simulink model "rc_filter_test"  (R2020b)
settings: Solver=VariableStepAuto  StartTime=0.0  StopTime=10.0  RelTol=1e-3
undefined symbols (not defined in the file): C, current_gain, R, R_load, R_sense
libraries: fl_lib x7, nesl_utility x4, ee_lib x1
settings Model: Creator=akern  LastModifiedBy=akern

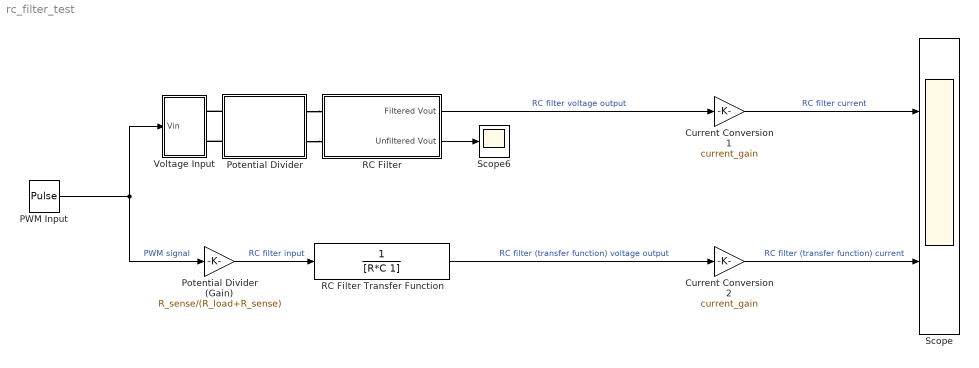
== system rc_filter_test ==
  Current Conversion 1 : Gain  Gain=current_gain
  Current Conversion 2 : Gain  Gain=current_gain
  PWM Input : DiscretePulseGenerator  PulseType=Time based  Amplitude=5  Period=1/500  PulseWidth=50
  Potential Divider : Subsystem
  Potential Divider (Gain) : Gain  Gain=R_sense/(R_load+R_sense)
  RC Filter : Subsystem
  RC Filter Transfer Function : TransferFcn  Numerator=[0 1]  Denominator=[R*C 1]
  Scope : Scope  NumInputPorts=2
  Scope6 : Scope
  Voltage Input : Subsystem
  wires:
  Current Conversion 1/1 -> Scope/1  "RC filter current"
  RC Filter/1(Filtered Vout) -> Current Conversion 1/1  "RC filter voltage output"
  RC Filter Transfer Function/1 -> Current Conversion 2/1  "RC filter (transfer function) voltage output"
  Potential Divider (Gain)/1 -> RC Filter Transfer Function/1  "RC filter input"
  PWM Input/1 -> Potential Divider (Gain)/1, Voltage Input/1(Vin)  "PWM signal"
  Current Conversion 2/1 -> Scope/2  "RC filter (transfer function) current"
  RC Filter/2(Unfiltered Vout) -> Scope6/1
  connections:
  Potential Divider/RConn2 -- RC Filter/LConn2
  Potential Divider/LConn2 -- Voltage Input/RConn2
  Potential Divider/LConn1 -- Voltage Input/RConn1
  Potential Divider/RConn1 -- RC Filter/LConn1

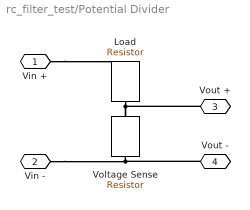
== system rc_filter_test/Potential Divider ==
  Load : fl_lib/Electrical/Electrical Elements/Resistor  R=R_load Ohm  i_specify=off  i_priority=None  i=0 A  i_nominal_specify=off  i_nominal_unit=A  i_nominal_value=1  v_specify=off  v_priority=None  v=0 V  v_nominal_specify=off  v_nominal_unit=V  v_nominal_value=1
  Voltage Sense : fl_lib/Electrical/Electrical Elements/Resistor  R=1 Ohm  i_specify=off  i_priority=None  i=0 A  i_nominal_specify=off  i_nominal_unit=A  i_nominal_value=1  v_specify=off  v_priority=None  v=0 V  v_nominal_specify=off  v_nominal_unit=V  v_nominal_value=1
  Vin + : PMIOPort  Side=Left
  Vin - : PMIOPort  Port=2  Side=Left
  Vout + : PMIOPort  Port=3  Side=Right
  Vout - : PMIOPort  Port=4  Side=Right
  connections:
  Vin +/RConn1 -- Load/LConn1
  Load/RConn1 -- Voltage Sense/LConn1 -- Vout +/RConn1
  Vin -/RConn1 -- Voltage Sense/RConn1 -- Vout -/RConn1

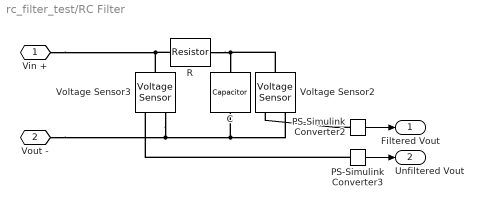
== system rc_filter_test/RC Filter ==
  C : ee_lib/Passive/Capacitor  cap_option=0  c=C F  Cvec=[1e-05, 1e-06] F  Vvec=[0, 10] V  CV_table_symmetry=1  f_vec=[1, 10] kHz  DFext_vec=[.8, 1.2]  C_tol=5  enable_C_tol=0  tol_distribution=1  nSigma=4  r=1e-6 Ohm  g=0 1/Ohm  averaging_period=0 s  enable_operating_limits=0  operating_limit_action=2  max_working_voltage_range=[-25, 25] V  power_rating=1 W  enable_faults=0  fault_action=1  Cscale_faulted=100  R_faulted=1e-3 Ohm  G_faulted=0 1/Ohm  tau_fault=1e-3 s  enable_temporal_fault=0  t_fault=1 s  enable_behavioral_fault=0  max_permissible_voltage_range=[-100, 100] V  t_fail_on_voltage=1 s  i_specify=off  i_priority=None  i=0 A  i_nominal_specify=off  i_nominal_unit=A  i_nominal_value=1  v_specify=off  v_priority=None  v=0 V  v_nominal_specify=off  v_nominal_unit=V  v_nominal_value=1  vc_specify=off  vc_priority=High  vc=0 V  vc_nominal_specify=off  vc_nominal_unit=V  vc_nominal_value=1
  PS-Simulink Converter2 : nesl_utility/PS-Simulink Converter  PhysicalDomain=network_engine_domain  SubClassName=ps_output  LeftPortType=input  RightPortType=output  PseudoPeriodic=off  Frequencies=[]  Unit=inherit  AffineConversion=off
  PS-Simulink Converter3 : nesl_utility/PS-Simulink Converter  PhysicalDomain=network_engine_domain  SubClassName=ps_output  LeftPortType=input  RightPortType=output  PseudoPeriodic=off  Frequencies=[]  Unit=inherit  AffineConversion=off
  R : fl_lib/Electrical/Electrical Elements/Resistor  R=R Ohm  i_specify=off  i_priority=None  i=0 A  i_nominal_specify=off  i_nominal_unit=A  i_nominal_value=1  v_specify=off  v_priority=None  v=0 V  v_nominal_specify=off  v_nominal_unit=V  v_nominal_value=1
  Voltage Sensor2 : fl_lib/Electrical/Electrical Sensors/Voltage Sensor
  Voltage Sensor3 : fl_lib/Electrical/Electrical Sensors/Voltage Sensor
  Vin + : PMIOPort  Side=Left
  Vout - : PMIOPort  Port=2  Side=Left
  Filtered Vout : Outport
  Unfiltered Vout : Outport  Port=2
  wires:
  PS-Simulink Converter2/1 -> Filtered Vout/1
  PS-Simulink Converter3/1 -> Unfiltered Vout/1
  connections:
  Voltage Sensor3/RConn2 -- C/RConn1 -- Voltage Sensor2/RConn2 -- Vout -/RConn1
  R/RConn1 -- C/LConn1 -- Voltage Sensor2/LConn1
  Voltage Sensor3/LConn1 -- R/LConn1 -- Vin +/RConn1
  PS-Simulink Converter3/LConn1 -- Voltage Sensor3/RConn1
  PS-Simulink Converter2/LConn1 -- Voltage Sensor2/RConn1

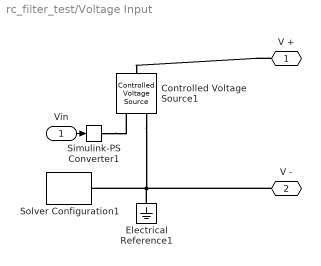
== system rc_filter_test/Voltage Input ==
  Vin : Inport
  Controlled Voltage Source1 : fl_lib/Electrical/Electrical Sources/Controlled Voltage Source
  Electrical Reference1 : fl_lib/Electrical/Electrical Elements/Electrical Reference
  Simulink-PS Converter1 : nesl_utility/Simulink-PS Converter  PhysicalDomain=network_engine_domain  SubClassName=ps_input  LeftPortType=input  RightPortType=output  PseudoPeriodic=off  Frequencies=[]  NoiseDistribution=none  NoiseParameters=[]  Unit=1  AffineConversion=off  FilteringAndDerivatives=provide  SimscapeFilterOrder=1  InputFilterTimeConstant=0.001  UdotUserProvided=0
  Solver Configuration1 : nesl_utility/Solver Configuration  PhysicalDomain=network_engine_domain  SubClassName=solver  LeftPortType=input  RightPortType=generic  Tones=[]  Harmonics=[]  SimulateNoise=off  Profile=off  UseLocalSampling=off  EnableSwitchedLinearOptims=on  FrequencyDomain=off  UseCCode=off  RelTol=0.001  AbsTol=1e-06  MinStep=1e-09  ToWorkspace=off  RevertToSquareIcSolve=off  NumHomotopyIterations=100  PhasorMode=off  PhasorModeNumHarmonics=1  DoDC=off  ResidualTolerance=1e-09  UseLocalSolver=off  LocalSolverChoice=NE_BACKWARD_EULER_ADVANCER  LocalSolverSampleTime=0.001  DoFixedCost=off  MaxNonlinIter=3  MaxModeIter=2  ComputeImpulses=off  ImpulseIterations=2  LinearAlgebra=auto  EquationFormulation=NE_TIME_EF  DelaysMemoryBudget=1024  AutomaticFiltering=on  FilteringTimeConstant=0.001  PartitionStorageMethod=AS_NEEDED  PartitionMemoryBudget=1024  PartitionMethod=ROBUST
  V + : PMIOPort  Side=Right
  V - : PMIOPort  Port=2  Side=Right
  wires:
  Vin/1 -> Simulink-PS Converter1/1
  connections:
  Simulink-PS Converter1/RConn1 -- Controlled Voltage Source1/RConn1
  V +/RConn1 -- Controlled Voltage Source1/LConn1
  Controlled Voltage Source1/RConn2 -- Electrical Reference1/LConn1 -- Solver Configuration1/RConn1 -- V -/RConn1
